simulink model "Problem2"  (R2025b)
settings: Solver=VariableStepAuto  StartTime=0.0  StopTime=10.0  RelTol=1e-3
settings Model: Creator=hp  LastModifiedBy=hp

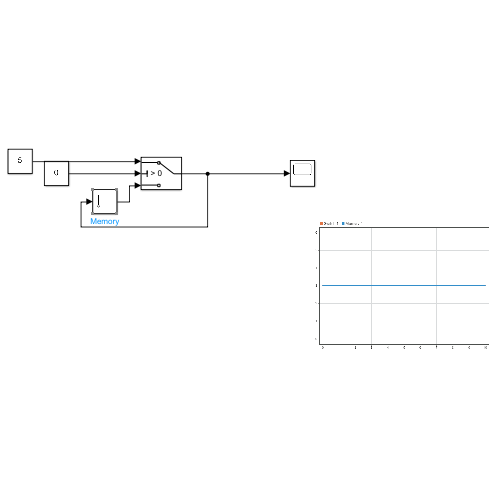
[thumbnail: Simulink's stored preview of the top-level diagram]
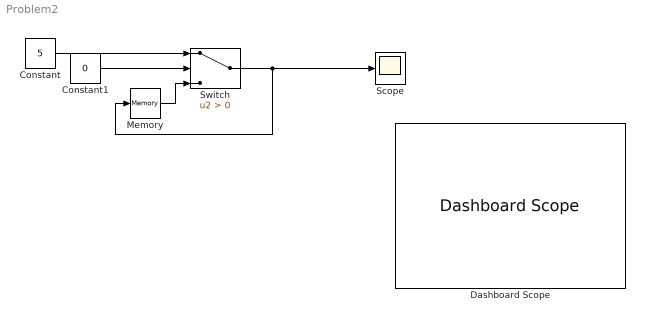
== system Problem2 ==
  Constant : Constant  Value=5
  Constant1 : Constant  Value=0
  Dashboard Scope : DashboardScope  FontColor=[0.0, 0.0, 0.0]
  Memory : Memory  InitialCondition=3
  Scope : Scope
      settings: ActiveDisplayYMinimum=2  ActiveDisplayYMaximum=4
  Switch : Switch  Criteria=u2 > Threshold  SaturateOnIntegerOverflow=off  InputSameDT=off
  wires:
  Constant1/1 -> Switch/2
  Constant/1 -> Switch/1
  Switch/1 -> Memory/1, Scope/1
  Memory/1 -> Switch/3
